simulink model "sg_2d_fir"  (Simulink 7.6)
settings: Solver=ode45  StartTime=0.0  StopTime=1600.0  RelTol=1e-3
undefined symbols (not defined in the file): gcbh, xlBlockLoadCallback, xlGetNormalizedPeriod, xlipgetpartsetting
libraries: xbsIndex_r4 x311, dspsrcs4 x6
(part 1 of 4)
settings Model: Creator=tbooth  LastModifiedBy=tawassne
settings OptimizationCC: InitFltsAndDblsToZero=on
settings DebuggingCC: SaveWithParameterizedLinksMsg=none  SignalResolutionControl=TryResolveAllWithWarning  MultiTaskDSMMsg=warning  MultiTaskCondExecSysMsg=none  StrictBusMsg=Warning
settings RTWCC: IncludeERTFirstTime=on
settings GRTTargetCC: TargetFcnLib=ansi_tfl_tmw.mat

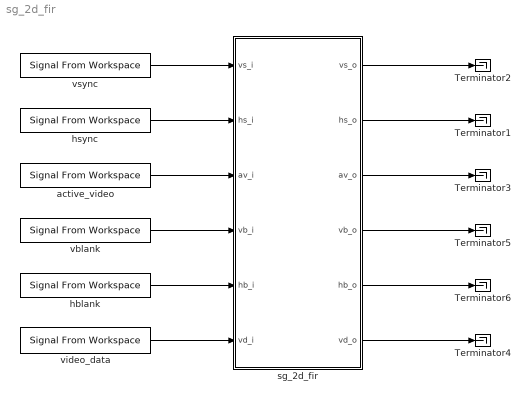
== system sg_2d_fir ==
  Terminator{1..6} (6 alike) : Terminator
  active_video : dspsrcs4/Signal From Workspace  SystemSampleTime=-1  X="[ones(1,90) zeros(1,10)  ]"  Ts=1  nsamps=1  OutputAfterFinalValue=Cyclic repetition  ignoreOrWarnInputAndFrameLengths=off
  hblank : dspsrcs4/Signal From Workspace  SystemSampleTime=-1  X=[ zeros(1,1) ones(1,99) ]  Ts=1  nsamps=1  OutputAfterFinalValue=Cyclic repetition  ignoreOrWarnInputAndFrameLengths=off
  hsync : dspsrcs4/Signal From Workspace  SystemSampleTime=-1  X=[ zeros(1,1) ones(1,99) ]  Ts=1  nsamps=1  OutputAfterFinalValue=Cyclic repetition  ignoreOrWarnInputAndFrameLengths=off
  sg_2d_fir : Subsystem
  vblank : dspsrcs4/Signal From Workspace  SystemSampleTime=-1  X=[ zeros(1,100) ones(1,900) ]  Ts=1  nsamps=1  OutputAfterFinalValue=Cyclic repetition  ignoreOrWarnInputAndFrameLengths=off
  video_data : dspsrcs4/Signal From Workspace  SystemSampleTime=-1  X=[repmat([10, 20],1,40),zeros(1,20), repmat([20,15],1,40) ,zeros(1,20)]  Ts=1  nsamps=1  OutputAfterFinalValue=Cyclic repetition  ignoreOrWarnInputAndFrameLengths=off
      link override From Workspace: OutputAfterFinalValue=Cyclic repetition
  vsync : dspsrcs4/Signal From Workspace  SystemSampleTime=-1  X=[ zeros(1,100) ones(1,900) ]  Ts=1  nsamps=1  OutputAfterFinalValue=Cyclic repetition  ignoreOrWarnInputAndFrameLengths=off
  wires:
  vsync/1 -> sg_2d_fir/1(vs_i)
  hsync/1 -> sg_2d_fir/2(hs_i)
  active_video/1 -> sg_2d_fir/3(av_i)
  sg_2d_fir/1(vs_o) -> Terminator2/1
  sg_2d_fir/2(hs_o) -> Terminator1/1
  sg_2d_fir/3(av_o) -> Terminator3/1
  sg_2d_fir/6(vd_o) -> Terminator4/1
  video_data/1 -> sg_2d_fir/6(vd_i)
  vblank/1 -> sg_2d_fir/4(vb_i)
  hblank/1 -> sg_2d_fir/5(hb_i)
  sg_2d_fir/4(vb_o) -> Terminator5/1
  sg_2d_fir/5(hb_o) -> Terminator6/1

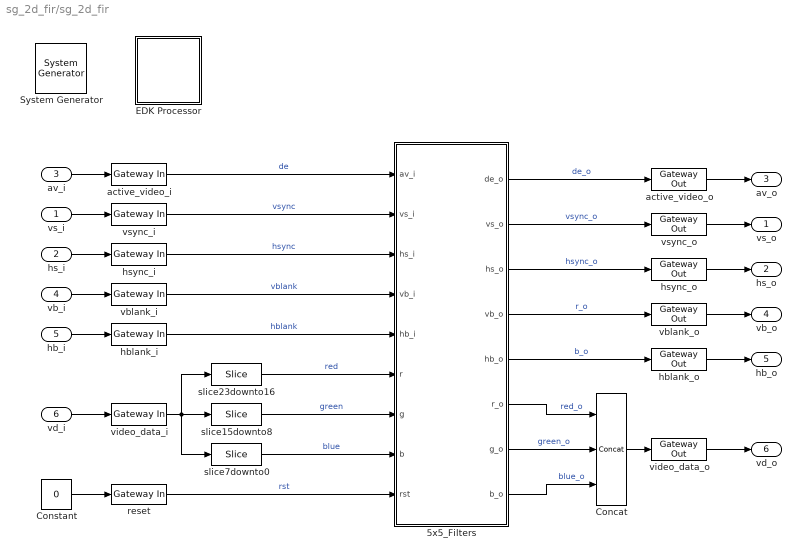
== system sg_2d_fir/sg_2d_fir ==
  vs_i : Inport
  hs_i : Inport  Port=2
  av_i : Inport  Port=3
  vb_i : Inport  Port=4
  hb_i : Inport  Port=5
  vd_i : Inport  Port=6
  " System Generator" : xbsIndex_r4/ System Generator  Tag=genX  SystemSampleTime=-1  xilinxfamily=spartan6  part=xc6slx150t  speed=-3  package=fgg676  synthesis_tool=XST  clock_wrapper=Clock Enables  directory=./sg_rgb_2d_fir_s6  proj_type=Project Navigator  Synth_file=XST Defaults  Impl_file=ISE Defaults  testbench=off  simulink_period=1  sysclk_period=10  dcm_input_clock_period=10  incr_netlist=off  trim_vbits=Everywhere in SubSystem  dbl_ovrd=According to Block Masks  core_generation=According to Block Masks  run_coregen=off  deprecated_control=off  eval_field=0  block_type=sysgen
      settings: block_version=11.4
  5x5_Filters : Subsystem
  Concat : xbsIndex_r4/Concat  num_inputs=3  dbl_ovrd=off  block_type=concat
  Constant : Constant  Value=0
  EDK Processor : Subsystem  LoadFcn=xlBlockLoadCallback(gcbh);  mask(Xilinx EDK Processor Block){mode=EDK pcore generation, xmp=, MemVisToProc=<qt bgcolor="#FFFFFF"><div><img src="C:/Program_Waj/Xilinx_13.1/ISE_DS/ISE/sysgen/data/images/registerminus.gif"> &lt;&lt;coef_update&gt;&gt;<br> <img src="C:/Program_Waj/Xilinx_13.1/ISE_DS/ISE/sysgen/data/images/parameters.gif"> Type : Fix_1_0<br> <img src="C:/Program_Waj/Xilinx_13.1/ISE_DS/ISE/sysgen/data/images/parameters.gif"> Addr : 0x80000800<br></div><div><img src="C:/Program_Waj/Xilinx_13.1/ISE_DS/ISE/sysgen/data/images/registerminus.gif"> &lt;&lt;coef_gain&gt;&gt;<br> <img src="C:/Program_Waj/Xilinx_13.1/ISE_DS/ISE/sysgen/data/images/parameters.gif"> Type : Fix_20_17<br> <img src="C:/Program_Waj/Xilinx_13.1/ISE_DS/ISE/sysgen/data/images/parameters.gif"> Addr : 0x80000804<br></div><div><img src="C:/Program_Waj/Xilinx_13.1/ISE_DS/ISE/sysgen/data/images/memoryminus.gif"> &lt;&lt;coef_buffer&gt;&gt;<br> <img src="C:/Program_Waj/Xilinx_13.1/ISE_DS/ISE/sysgen/data/images/parameters.gif"> Type : Fix_7_0<br> <img src="C:/Program_Waj/Xilinx_13.1/ISE_DS/ISE/sysgen/data/images/parameters.gif"> Addr : 0x80000000<br> <img src="C:/Program_Waj/Xilinx_13.1/ISE_DS/ISE/sysgen/data/images/parameters.gif"> Depth : 32<br></div></qt>, AvailableMemories=<empty>, portInterfaceTable={'exposed'=>[],'portdir'=>[],'portname'=>[],'shortname'=>[]}, bus_type_sgadvanced=, bus_type=PLB, baseaddr=0x80000000, baseaddr_lock_sgadvanced=, baseaddr_lock=off, dual_clock_sgadvanced=, dual_clock=on, reg_readback_sgadvanced=, reg_readback=on, ucf_file=, inheritDeviceType_sgadvanced=, inheritDeviceType=off, elf_file=, codebug_sgadvanced=, codebug=on, clock_name=plb, internalPortList={}, resetPolarity=0, memxtable={'mladdr'=>[0.00000000000000000,1.00000000000000000,-1.00000000000000000],'mlist'=>['sg_2d_fir/sg_2d_fir/5x5_Filters/coefficient_memory/From Register1','sg_2d_fir/sg_2d_fir/5x5_Filters/coefficient_memory/From Register','sg_2d_fir/sg_2d_fir/5x5_Filters/coefficient_memory/Shared Memory'],'mlname'=>['\\'coef_update\\'','\\'coef_gain\\'','\\'coef_buffer\\''],'mlstate'=>[1.00000000000000000,1.00000000000000000,1.00000000000000000]}, procinfo={}, memmapdirty=off, blockname=, xpsintstyle=default, has_advanced_control=0, sggui_pos=595,80,379,436, block_type=edkprocessor, block_version=2.7, sg_icon_stat=62,64,-1,-1,white,blue,0,07734,right,,[ ],[ ], sg_mask_display=|, sg_list_contents={'table'=>{'AvailableMemories'=>'popup(<empty>)'}}, sg_blockgui_xml=}
      mask sg_mask_display=|
      | fprintf('','COMMENT: begin icon graphics');
      | patch([0 62 62 0 0 ],[0 0 64 64 0 ],[0.77 0.82 0.91 ]);
      | plot([0 62 62 0 0 ],[0 0 64 64 0 ]);
      | patch([13.2 24.76 32.76 40.76 48.76 32.76 21.2 13.2 ],[40.88 40.88 48.88 40.88 48.88 48.88 48.88 40.88 ],[1 1 1 ]);
      | patch([21.2 32.76 24.76 13.2 21.2 ],[32.88 32.88 40.88 40.88 32.88 ],[0.931 0.946 0.973 ]);
      | patch([13.2 24.76 32.76 21.2 13.2 ],[24.88 24.88 32.88 32.88 24.88 ],[1 1 1 ]);
      | patch([21.2 48.76 40.76 32.76 24.76 13.2 21.2 ],[16.88 16.88 24.88 16.88 24.88 24.88 16.88 ],[0.931 0.946 0.973 ]);
      | fprintf('','COMMENT: end icon graphics');
      | fprintf('','COMMENT: begin icon text');
      | fprintf('','COMMENT: end icon text');
      mask prompts: mode "Configure Processor for"; xmp "XPS Project"; MemVisToProc ""; AvailableMemories "Available Memories"; portInterfaceTable ""; bus_type_sgadvanced ""; bus_type "Bus Type"; baseaddr "Base Address"; baseaddr_lock_sgadvanced ""; baseaddr_lock "Lock"; dual_clock_sgadvanced ""; dual_clock "Dual Clocks"; reg_readback_sgadvanced ""; reg_readback "Register Read-Back"; ucf_file "Constraint File"; inheritDeviceType_sgadvanced ""; inheritDeviceType "Inherit Device Type"; elf_file "Initial Program"; codebug_sgadvanced ""; codebug "Enable Co-Debug with Xilinx SDK (Beta)"; clock_name ""; internalPortList ""; resetPolarity ""; memxtable ""; procinfo ""; memmapdirty ""; blockname ""; xpsintstyle ""; has_advanced_control ""; sggui_pos ""; block_type ""; block_version ""; sg_icon_stat ""; sg_mask_display ""; sg_list_contents ""; sg_blockgui_xml ""
      mask help: Xilinx EDK Processor
      mask init:
      | try
      |   tmp_gcb = gcb;
      |   tmp_gcbh = gcbh;
      |   if (strcmp('SysGenIndex',get_param(bdroot(tmp_gcbh),'tag')) && ~isempty(regexp(bdroot(tmp_gcb), '^xbs', 'once')))
      |     return;
      |   end;
      |   xlMungeMaskParams;
      | 
      |   block_type='edkprocessor';
      | 
      |   serialized_declarations = '{''block_type''=>''String''}';
      |   xledkprocessor_init();
      |   ptable_ = xlblockprep(get_param(tmp_gcb, 'MaskWSVariables'));
      |   try
      |     xlBlockMoveCallback(tmp_gcbh);
      |   catch 
      |      clear global xl_updateicon_recursion_guard;
      |   end;
      | catch
      |   global dbgsysgen;
      |   if(~isempty(dbgsysgen) && dbgsysgen)
      |     e = regexprep(lasterr, '\n', '\nError: ');
      |     disp(['Error: While running MaskInit code on block ' tmp_gcb ': ' e]);
      |     error(e);
      |   end
      | end
      settings: CopyFcn=xlProcBlockCopyCallback(gcbh);xlBlockMoveCallback(gcbh);  DeleteFcn=xlDestroyGui(gcbh);  ModelCloseFcn=xlDestroyGui(gcbh);  PreSaveFcn=xlBlockPreSaveCallback(gcbh);  PostSaveFcn=xlBlockPostSaveCallback(gcbh);  DestroyFcn=xlDestroyGui(gcbh);  OpenFcn=bh=gcbh;xlProcBlockCallbacks('populatesharedmemorylistbox',bh);xlOpenGui(bh, 'edkprocessor_gui.xml', @xlProcBlockEnablement, @xlProcBlockAction);  CloseFcn=xlDestroyGui(gcbh);  MoveFcn=xlBlockMoveCallback(gcbh);
      mask Help: eval('');xlDoc('-book','sysgen','-topic','EDK_Processor');
      mask StyleString: popup(EDK pcore generation|HDL netlisting),edit,edit,edit,edit,edit,popup(AXI|PLB),edit,edit,checkbox,edit,checkbox,edit,checkbox,edit,edit,checkbox,edit,edit,checkbox,edit,edit,edit,edit,edit,edit,edit,edit,edit,edit,edit,edit,edit,edit,edit,edit
      mask Display:
      | fprintf('','COMMENT: begin icon graphics');
      | patch([0 62 62 0 0 ],[0 0 64 64 0 ],[0.77 0.82 0.91 ]);
      | plot([0 62 62 0 0 ],[0 0 64 64 0 ]);
      | patch([13.2 24.76 32.76 40.76 48.76 32.76 21.2 13.2 ],[40.88 40.88 48.88 40.88 48.88 48.88 48.88 40.88 ],[1 1 1 ]);
      | patch([21.2 32.76 24.76 13.2 21.2 ],[32.88 32.88 40.88 40.88 32.88 ],[0.931 0.946 0.973 ]);
      | patch([13.2 24.76 32.76 21.2 13.2 ],[24.88 24.88 32.88 32.88 24.88 ],[1 1 1 ]);
      | patch([21.2 48.76 40.76 32.76 24.76 13.2 21.2 ],[16.88 16.88 24.88 16.88 24.88 24.88 16.88 ],[0.931 0.946 0.973 ]);
      | fprintf('','COMMENT: end icon graphics');
      | fprintf('','COMMENT: begin icon text');
      | disp('');
      | 
      | fprintf('','COMMENT: end icon text');
  active_video_i : xbsIndex_r4/Gateway In  gui_display_data_type=Fixed-point  arith_type=Unsigned  n_bits=1  bin_pt=0  preci_type=Single  exp_width=8  frac_width=24  quantization="Round  (unbiased: +/- Inf)"  overflow=Saturate  period=1  dbl_ovrd=off  timing_constraint=None  locs_specified=off  LOCs={}  hdl_port=on  block_type=gatewayin
      settings: infoedit="Gateway in block.  Converts inputs of type Simulink integer, double and fixed point to  Xilinx fixed point type.<P><P>Hardware notes:  In hardware these blocks become top level input ports."  xl_area=[0, 0, 0, 0, 0, 0, 0]  block_version=VER_STRING_GOES_HERE
  active_video_o : xbsIndex_r4/Gateway Out  hdl_port=on  timing_constraint=None  locs_specified=off  LOCs={}  block_type=gatewayout
      settings: infoedit="Gateway out block.  Converts Xilinx fixed point inputs into ouputs of type Simulink integer, double, or fixed point.<P><P>Hardware notes:  In hardware these blocks become top level output ports or are discarded, depending on how they are configured."  xl_area=[0, 0, 0, 0, 0, 0, 0]  block_version=VER_STRING_GOES_HERE
  hblank_i : xbsIndex_r4/Gateway In  gui_display_data_type=Fixed-point  arith_type=Unsigned  n_bits=1  bin_pt=0  preci_type=Single  exp_width=8  frac_width=24  quantization="Round  (unbiased: +/- Inf)"  overflow=Saturate  period=1  dbl_ovrd=off  timing_constraint=None  locs_specified=off  LOCs={}  hdl_port=on  block_type=gatewayin
      settings: infoedit="Gateway in block.  Converts inputs of type Simulink integer, double and fixed point to  Xilinx fixed point type.<P><P>Hardware notes:  In hardware these blocks become top level input ports."  xl_area=[0, 0, 0, 0, 0, 0, 0]  block_version=VER_STRING_GOES_HERE
  hblank_o : xbsIndex_r4/Gateway Out  hdl_port=on  timing_constraint=None  locs_specified=off  LOCs={}  block_type=gatewayout
      settings: infoedit="Gateway out block.  Converts Xilinx fixed point inputs into ouputs of type Simulink integer, double, or fixed point.<P><P>Hardware notes:  In hardware these blocks become top level output ports or are discarded, depending on how they are configured."  xl_area=[0, 0, 0, 0, 0, 0, 0]  block_version=VER_STRING_GOES_HERE
  hsync_i : xbsIndex_r4/Gateway In  gui_display_data_type=Fixed-point  arith_type=Unsigned  n_bits=1  bin_pt=0  preci_type=Single  exp_width=8  frac_width=24  quantization="Round  (unbiased: +/- Inf)"  overflow=Saturate  period=1  dbl_ovrd=off  timing_constraint=None  locs_specified=off  LOCs={}  hdl_port=on  block_type=gatewayin
      settings: infoedit="Gateway in block.  Converts inputs of type Simulink integer, double and fixed point to  Xilinx fixed point type.<P><P>Hardware notes:  In hardware these blocks become top level input ports."  xl_area=[0, 0, 0, 0, 0, 0, 0]  block_version=VER_STRING_GOES_HERE
  hsync_o : xbsIndex_r4/Gateway Out  hdl_port=on  timing_constraint=None  locs_specified=off  LOCs={}  block_type=gatewayout
      settings: infoedit="Gateway out block.  Converts Xilinx fixed point inputs into ouputs of type Simulink integer, double, or fixed point.<P><P>Hardware notes:  In hardware these blocks become top level output ports or are discarded, depending on how they are configured."  xl_area=[0, 0, 0, 0, 0, 0, 0]  block_version=VER_STRING_GOES_HERE
  reset : xbsIndex_r4/Gateway In  gui_display_data_type=Fixed-point  arith_type=Unsigned  n_bits=1  bin_pt=0  preci_type=Single  exp_width=8  frac_width=24  quantization="Round  (unbiased: +/- Inf)"  overflow=Saturate  period=1  dbl_ovrd=off  timing_constraint=None  locs_specified=off  LOCs={}  hdl_port=on  block_type=gatewayin
      settings: infoedit="Gateway in block.  Converts inputs of type Simulink integer, double and fixed point to  Xilinx fixed point type.<P><P>Hardware notes:  In hardware these blocks become top level input ports."
  slice15downto8 : xbsIndex_r4/Slice  nbits=8  boolean_output=off  mode=Lower Bit Location + Width  bit1=0  base1=MSB of Input  bit0=8  base0=LSB of Input  dbl_ovrd=off  block_type=slice
  slice23downto16 : xbsIndex_r4/Slice  nbits=8  boolean_output=off  mode=Lower Bit Location + Width  bit1=0  base1=MSB of Input  bit0=16  base0=LSB of Input  dbl_ovrd=off  block_type=slice
  slice7downto0 : xbsIndex_r4/Slice  nbits=8  boolean_output=off  mode=Lower Bit Location + Width  bit1=0  base1=MSB of Input  bit0=0  base0=LSB of Input  dbl_ovrd=off  block_type=slice
  vblank_i : xbsIndex_r4/Gateway In  gui_display_data_type=Fixed-point  arith_type=Unsigned  n_bits=1  bin_pt=0  preci_type=Single  exp_width=8  frac_width=24  quantization="Round  (unbiased: +/- Inf)"  overflow=Saturate  period=1  dbl_ovrd=off  timing_constraint=None  locs_specified=off  LOCs={}  hdl_port=on  block_type=gatewayin
      settings: infoedit="Gateway in block.  Converts inputs of type Simulink integer, double and fixed point to  Xilinx fixed point type.<P><P>Hardware notes:  In hardware these blocks become top level input ports."  xl_area=[0, 0, 0, 0, 0, 0, 0]  block_version=VER_STRING_GOES_HERE
  vblank_o : xbsIndex_r4/Gateway Out  hdl_port=on  timing_constraint=None  locs_specified=off  LOCs={}  block_type=gatewayout
      settings: infoedit="Gateway out block.  Converts Xilinx fixed point inputs into ouputs of type Simulink integer, double, or fixed point.<P><P>Hardware notes:  In hardware these blocks become top level output ports or are discarded, depending on how they are configured."  xl_area=[0, 0, 0, 0, 0, 0, 0]  block_version=VER_STRING_GOES_HERE
  video_data_i : xbsIndex_r4/Gateway In  gui_display_data_type=Fixed-point  arith_type=Unsigned  n_bits=24  bin_pt=0  preci_type=Single  exp_width=8  frac_width=24  quantization="Round  (unbiased: +/- Inf)"  overflow=Saturate  period=1  dbl_ovrd=off  timing_constraint=None  locs_specified=off  LOCs={}  hdl_port=on  block_type=gatewayin
      settings: infoedit="Gateway in block.  Converts inputs of type Simulink integer, double and fixed point to  Xilinx fixed point type.<br><br>Hardware notes:  In hardware these blocks become top level input ports."  xl_area=[0, 0, 0, 0, 0, 0, 0]  block_version=VER_STRING_GOES_HERE
  video_data_o : xbsIndex_r4/Gateway Out  hdl_port=on  timing_constraint=None  locs_specified=off  LOCs={}  block_type=gatewayout
      settings: infoedit="Gateway out block.  Converts Xilinx fixed point inputs into ouputs of type Simulink integer, double, or fixed point.<P><P>Hardware notes:  In hardware these blocks become top level output ports or are discarded, depending on how they are configured."  xl_area=[0, 0, 0, 0, 0, 0, 0]  block_version=VER_STRING_GOES_HERE
  vsync_i : xbsIndex_r4/Gateway In  gui_display_data_type=Fixed-point  arith_type=Unsigned  n_bits=1  bin_pt=0  preci_type=Single  exp_width=8  frac_width=24  quantization="Round  (unbiased: +/- Inf)"  overflow=Saturate  period=1  dbl_ovrd=off  timing_constraint=None  locs_specified=off  LOCs={}  hdl_port=on  block_type=gatewayin
      settings: infoedit="Gateway in block.  Converts inputs of type Simulink integer, double and fixed point to  Xilinx fixed point type.<P><P>Hardware notes:  In hardware these blocks become top level input ports."  xl_area=[0, 0, 0, 0, 0, 0, 0]  block_version=VER_STRING_GOES_HERE
  vsync_o : xbsIndex_r4/Gateway Out  hdl_port=on  timing_constraint=None  locs_specified=off  LOCs={}  block_type=gatewayout
      settings: infoedit="Gateway out block.  Converts Xilinx fixed point inputs into ouputs of type Simulink integer, double, or fixed point.<P><P>Hardware notes:  In hardware these blocks become top level output ports or are discarded, depending on how they are configured."  xl_area=[0, 0, 0, 0, 0, 0, 0]  block_version=VER_STRING_GOES_HERE
  vs_o : Outport
  hs_o : Outport  Port=2
  av_o : Outport  Port=3
  vb_o : Outport  Port=4
  hb_o : Outport  Port=5
  vd_o : Outport  Port=6
  wires:
  5x5_Filters/1(de_o) -> active_video_o/1  "de_o"
  5x5_Filters/2(vs_o) -> vsync_o/1  "vsync_o"
  5x5_Filters/3(hs_o) -> hsync_o/1  "hsync_o"
  Constant/1 -> reset/1
  hsync_i/1 -> 5x5_Filters/3(hs_i)  "hsync"
  active_video_i/1 -> 5x5_Filters/1(av_i)  "de"
  vsync_i/1 -> 5x5_Filters/2(vs_i)  "vsync"
  av_i/1 -> active_video_i/1
  vs_i/1 -> vsync_i/1
  hs_i/1 -> hsync_i/1
  vd_i/1 -> video_data_i/1
  active_video_o/1 -> av_o/1
  vsync_o/1 -> vs_o/1
  hsync_o/1 -> hs_o/1
  video_data_o/1 -> vd_o/1
  Concat/1 -> video_data_o/1
  slice23downto16/1 -> 5x5_Filters/6(r)  "red"
  reset/1 -> 5x5_Filters/9(rst)  "rst"
  vblank_o/1 -> vb_o/1
  hblank_o/1 -> hb_o/1
  vb_i/1 -> vblank_i/1
  hb_i/1 -> hblank_i/1
  5x5_Filters/4(vb_o) -> vblank_o/1  "r_o"
  5x5_Filters/5(hb_o) -> hblank_o/1  "b_o"
  vblank_i/1 -> 5x5_Filters/4(vb_i)  "vblank"
  hblank_i/1 -> 5x5_Filters/5(hb_i)  "hblank"
  video_data_i/1 -> slice7downto0/1, slice23downto16/1, slice15downto8/1
  slice15downto8/1 -> 5x5_Filters/7(g)  "green"
  slice7downto0/1 -> 5x5_Filters/8(b)  "blue"
  5x5_Filters/7(g_o) -> Concat/2  "green_o"
  5x5_Filters/8(b_o) -> Concat/3  "blue_o"
  5x5_Filters/6(r_o) -> Concat/1  "red_o"

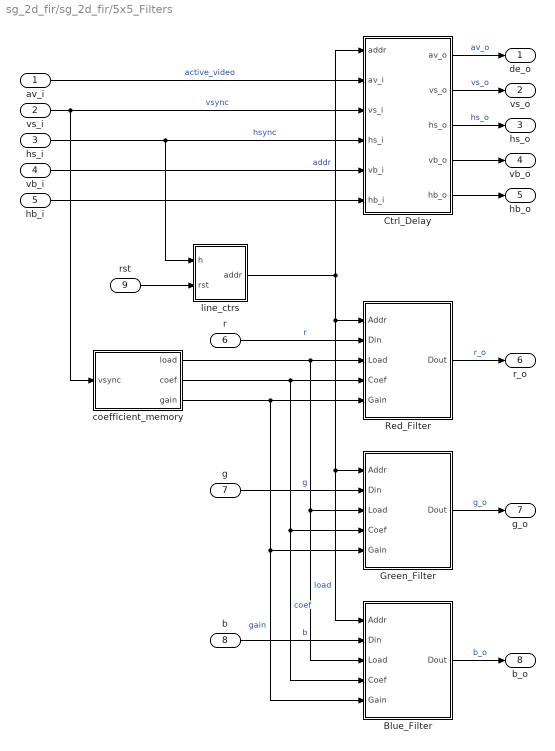
== system sg_2d_fir/sg_2d_fir/5x5_Filters ==
  av_i : Inport
  vs_i : Inport  Port=2
  hs_i : Inport  Port=3
  vb_i : Inport  Port=4
  hb_i : Inport  Port=5
  r : Inport  Port=6
  g : Inport  Port=7
  b : Inport  Port=8
  rst : Inport  Port=9
  Blue_Filter : Subsystem
  Ctrl_Delay : Subsystem
  Green_Filter : Subsystem
  Red_Filter : Subsystem
  coefficient_memory : Subsystem  mask{width=7, bin_pt=0, g_width=20, g_bin_pt=17, period=1}
      mask prompts: width "Coefficient Width"; bin_pt "Coefficient Binary Point"; g_width "Gain Width"; g_bin_pt "Gain Binary Point"; period "Sample Period"
      mask init:
      | %work around until plb initialization can use mask variables
      | 
      | c_width = sprintf('%d',width);
      | c_bin_pt = sprintf('%d',bin_pt);
      | c_g_width = sprintf('%d',g_width);
      | c_g_bin_pt = sprintf('%d',g_bin_pt);
      | 
      | blockPath = gcs;
      | set_param([blockPath '/coefficient_memory/Shared Memory'],'n_bits',c_width);
      | set_param([blockPath '/coefficient_memory/Shared Memory'],'bin_pt',c_bin_pt);
      | 
      | set_param([blockPath '/coefficient_memory/From Register'],'n_bits',c_g_width);
      | set_param([blockPath '/coefficient_memory/From Register'],'bin_pt',c_g_bin_pt);
  line_ctrs : Subsystem
  de_o : Outport
  vs_o : Outport  Port=2
  hs_o : Outport  Port=3
  vb_o : Outport  Port=4
  hb_o : Outport  Port=5
  r_o : Outport  Port=6
  g_o : Outport  Port=7
  b_o : Outport  Port=8
  wires:
  r/1 -> Red_Filter/2(Din)  "r"
  coefficient_memory/1(load) -> Red_Filter/3(Load), Green_Filter/3(Load), Blue_Filter/3(Load)  "load"
  coefficient_memory/2(coef) -> Red_Filter/4(Coef), Green_Filter/4(Coef), Blue_Filter/4(Coef)  "coef"
  Red_Filter/1(Dout) -> r_o/1  "r_o"
  coefficient_memory/3(gain) -> Red_Filter/5(Gain), Green_Filter/5(Gain), Blue_Filter/5(Gain)  "gain"
  hs_i/1 -> line_ctrs/1(h), Ctrl_Delay/4(hs_i)  "hsync"
  line_ctrs/1(addr) -> Ctrl_Delay/1(addr), Red_Filter/1(Addr), Green_Filter/1(Addr), Blue_Filter/1(Addr)  "addr"
  vs_i/1 -> Ctrl_Delay/3(vs_i), coefficient_memory/1(vsync)  "vsync"
  av_i/1 -> Ctrl_Delay/2(av_i)  "active_video"
  Ctrl_Delay/3(hs_o) -> hs_o/1  "hs_o"
  Ctrl_Delay/2(vs_o) -> vs_o/1  "vs_o"
  Ctrl_Delay/1(av_o) -> de_o/1  "av_o"
  g/1 -> Green_Filter/2(Din)  "g"
  Green_Filter/1(Dout) -> g_o/1  "g_o"
  b/1 -> Blue_Filter/2(Din)  "b"
  Blue_Filter/1(Dout) -> b_o/1  "b_o"
  rst/1 -> line_ctrs/2(rst)
  Ctrl_Delay/5(hb_o) -> hb_o/1
  Ctrl_Delay/4(vb_o) -> vb_o/1
  vb_i/1 -> Ctrl_Delay/5(vb_i)
  hb_i/1 -> Ctrl_Delay/6(hb_i)

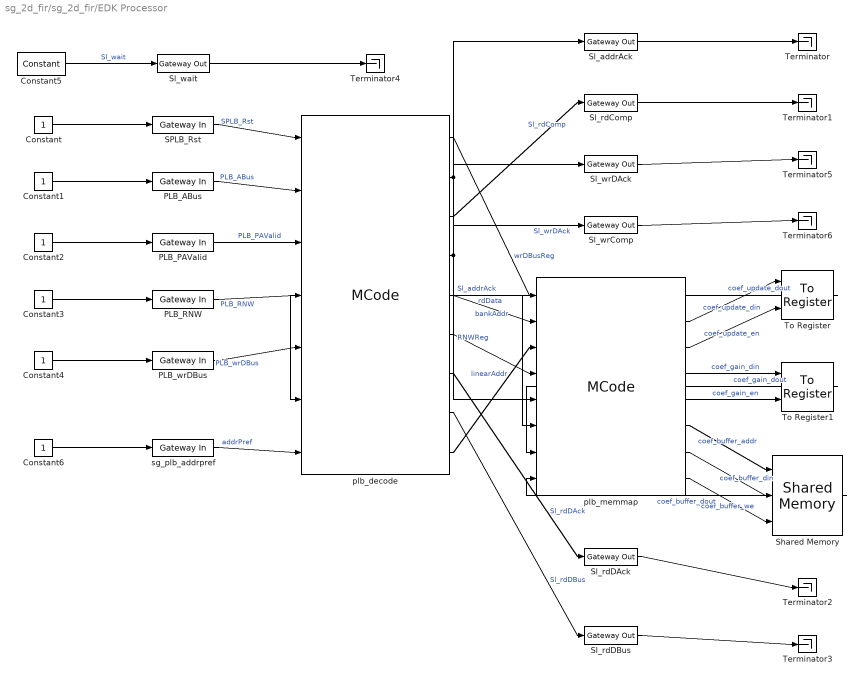
== system sg_2d_fir/sg_2d_fir/EDK Processor ==
  Constant{,1..4,6} (6 alike) : Constant
  Constant5 : xbsIndex_r4/Constant  const=0  gui_display_data_type=Fixed-point  arith_type=Unsigned  n_bits=1  bin_pt=0  preci_type=Single  exp_width=8  frac_width=24  explicit_period=on  period=xlGetNormalizedPeriod()  equ=P=C  opselect=C  inp2=PCIN>>17  opr=+  inp1=P  carry=CIN  dbl_ovrd=off  block_type=constant
  PLB_ABus : xbsIndex_r4/Gateway In  gui_display_data_type=Fixed-point  arith_type=Unsigned  n_bits=32  bin_pt=0  preci_type=Single  exp_width=8  frac_width=24  quantization="Round  (unbiased: +/- Inf)"  overflow=Saturate  period=xlGetNormalizedPeriod()  dbl_ovrd=off  timing_constraint=None  locs_specified=off  LOCs={}  hdl_port=on  block_type=gatewayin
      settings: infoedit="Gateway in block.  Converts inputs of type Simulink integer, double and fixed point to  Xilinx fixed point or floating-point data type.<br><br>Hardware notes:  In hardware these blocks become top level input ports."  sginterface={'Xilinx'=>{'jtaghwcosim'=>{'non_memory_mapped_port'=>'PLB_ABus'}},'iopad'=>{'constraint'=>'#'}}
  PLB_PAValid : xbsIndex_r4/Gateway In  gui_display_data_type=Fixed-point  arith_type=Unsigned  n_bits=1  bin_pt=0  preci_type=Single  exp_width=8  frac_width=24  quantization="Round  (unbiased: +/- Inf)"  overflow=Saturate  period=xlGetNormalizedPeriod()  dbl_ovrd=off  timing_constraint=None  locs_specified=off  LOCs={}  hdl_port=on  block_type=gatewayin
      settings: infoedit="Gateway in block.  Converts inputs of type Simulink integer, double and fixed point to  Xilinx fixed point or floating-point data type.<br><br>Hardware notes:  In hardware these blocks become top level input ports."  sginterface={'Xilinx'=>{'jtaghwcosim'=>{'non_memory_mapped_port'=>'PLB_PAValid'}},'iopad'=>{'constraint'=>'#'}}
  PLB_RNW : xbsIndex_r4/Gateway In  gui_display_data_type=Fixed-point  arith_type=Unsigned  n_bits=1  bin_pt=0  preci_type=Single  exp_width=8  frac_width=24  quantization="Round  (unbiased: +/- Inf)"  overflow=Saturate  period=xlGetNormalizedPeriod()  dbl_ovrd=off  timing_constraint=None  locs_specified=off  LOCs={}  hdl_port=on  block_type=gatewayin
      settings: infoedit="Gateway in block.  Converts inputs of type Simulink integer, double and fixed point to  Xilinx fixed point or floating-point data type.<br><br>Hardware notes:  In hardware these blocks become top level input ports."  sginterface={'Xilinx'=>{'jtaghwcosim'=>{'non_memory_mapped_port'=>'PLB_RNW'}},'iopad'=>{'constraint'=>'#'}}
  PLB_wrDBus : xbsIndex_r4/Gateway In  gui_display_data_type=Fixed-point  arith_type=Unsigned  n_bits=32  bin_pt=0  preci_type=Single  exp_width=8  frac_width=24  quantization="Round  (unbiased: +/- Inf)"  overflow=Saturate  period=xlGetNormalizedPeriod()  dbl_ovrd=off  timing_constraint=None  locs_specified=off  LOCs={}  hdl_port=on  block_type=gatewayin
      settings: infoedit="Gateway in block.  Converts inputs of type Simulink integer, double and fixed point to  Xilinx fixed point or floating-point data type.<br><br>Hardware notes:  In hardware these blocks become top level input ports."  sginterface={'Xilinx'=>{'jtaghwcosim'=>{'non_memory_mapped_port'=>'PLB_wrDBus'}},'iopad'=>{'constraint'=>'#'}}
  SPLB_Rst : xbsIndex_r4/Gateway In  gui_display_data_type=Fixed-point  arith_type=Unsigned  n_bits=1  bin_pt=0  preci_type=Single  exp_width=8  frac_width=24  quantization="Round  (unbiased: +/- Inf)"  overflow=Saturate  period=xlGetNormalizedPeriod()  dbl_ovrd=off  timing_constraint=None  locs_specified=off  LOCs={}  hdl_port=on  block_type=gatewayin
      settings: infoedit="Gateway in block.  Converts inputs of type Simulink integer, double and fixed point to  Xilinx fixed point or floating-point data type.<br><br>Hardware notes:  In hardware these blocks become top level input ports."  sginterface={'Xilinx'=>{'jtaghwcosim'=>{'non_memory_mapped_port'=>'SPLB_Rst'}},'iopad'=>{'constraint'=>'#'}}
  Shared Memory : xbsIndex_r4/Shared Memory  shared_memory_name='coef_buffer'  depth=32  ownership=Owned and Initialized Elsewhere  initVector=sin(pi*(0:15)/16)  en=off  mutex=Unprotected  mode=Read and Write  write_mode=Read Before Write  time_out=0  latency=1  explicit_data_type=off  gui_display_data_type=Fixed-point  arith_type="Signed  (2's comp)"  n_bits=7  bin_pt=0  preci_type=Single  implementation=Block RAM  use_rpm=off  block_type=shmem
      settings: AttributesFormatString=<< %<shared_memory_name> >>
  Sl_addrAck : xbsIndex_r4/Gateway Out  hdl_port=on  timing_constraint=None  locs_specified=off  LOCs={}  block_type=gatewayout
      settings: infoedit="Gateway out block.  Converts Xilinx fixed point or floating-point type inputs into ouputs of type Simulink integer, double, or fixed point.<br><br>Hardware notes:  In hardware these blocks become top level output ports or are discarded, depending on how they are configured."  sginterface={'Xilinx'=>{'jtaghwcosim'=>{'non_memory_mapped_port'=>'Sl_addrAck'}},'iopad'=>{'constraint'=>'#'}}
  Sl_rdComp : xbsIndex_r4/Gateway Out  hdl_port=on  timing_constraint=None  locs_specified=off  LOCs={}  block_type=gatewayout
      settings: infoedit="Gateway out block.  Converts Xilinx fixed point or floating-point type inputs into ouputs of type Simulink integer, double, or fixed point.<br><br>Hardware notes:  In hardware these blocks become top level output ports or are discarded, depending on how they are configured."  sginterface={'Xilinx'=>{'jtaghwcosim'=>{'non_memory_mapped_port'=>'Sl_rdComp'}},'iopad'=>{'constraint'=>'#'}}
  Sl_rdDAck : xbsIndex_r4/Gateway Out  hdl_port=on  timing_constraint=None  locs_specified=off  LOCs={}  block_type=gatewayout
      settings: infoedit="Gateway out block.  Converts Xilinx fixed point or floating-point type inputs into ouputs of type Simulink integer, double, or fixed point.<br><br>Hardware notes:  In hardware these blocks become top level output ports or are discarded, depending on how they are configured."  sginterface={'Xilinx'=>{'jtaghwcosim'=>{'non_memory_mapped_port'=>'Sl_rdDAck'}},'iopad'=>{'constraint'=>'#'}}
  Sl_rdDBus : xbsIndex_r4/Gateway Out  hdl_port=on  timing_constraint=None  locs_specified=off  LOCs={}  block_type=gatewayout
      settings: infoedit="Gateway out block.  Converts Xilinx fixed point or floating-point type inputs into ouputs of type Simulink integer, double, or fixed point.<br><br>Hardware notes:  In hardware these blocks become top level output ports or are discarded, depending on how they are configured."  sginterface={'Xilinx'=>{'jtaghwcosim'=>{'non_memory_mapped_port'=>'Sl_rdDBus'}},'iopad'=>{'constraint'=>'#'}}
  Sl_wait : xbsIndex_r4/Gateway Out  hdl_port=on  timing_constraint=None  locs_specified=off  LOCs={}  block_type=gatewayout
      settings: infoedit="Gateway out block.  Converts Xilinx fixed point or floating-point type inputs into ouputs of type Simulink integer, double, or fixed point.<br><br>Hardware notes:  In hardware these blocks become top level output ports or are discarded, depending on how they are configured."  sginterface={'Xilinx'=>{'jtaghwcosim'=>{'non_memory_mapped_port'=>'Sl_wait'}},'iopad'=>{'constraint'=>'#'}}
  Sl_wrComp : xbsIndex_r4/Gateway Out  hdl_port=on  timing_constraint=None  locs_specified=off  LOCs={}  block_type=gatewayout
      settings: infoedit="Gateway out block.  Converts Xilinx fixed point or floating-point type inputs into ouputs of type Simulink integer, double, or fixed point.<br><br>Hardware notes:  In hardware these blocks become top level output ports or are discarded, depending on how they are configured."  sginterface={'Xilinx'=>{'jtaghwcosim'=>{'non_memory_mapped_port'=>'Sl_wrComp'}},'iopad'=>{'constraint'=>'#'}}
  Sl_wrDAck : xbsIndex_r4/Gateway Out  hdl_port=on  timing_constraint=None  locs_specified=off  LOCs={}  block_type=gatewayout
      settings: infoedit="Gateway out block.  Converts Xilinx fixed point or floating-point type inputs into ouputs of type Simulink integer, double, or fixed point.<br><br>Hardware notes:  In hardware these blocks become top level output ports or are discarded, depending on how they are configured."  sginterface={'Xilinx'=>{'jtaghwcosim'=>{'non_memory_mapped_port'=>'Sl_wrDAck'}},'iopad'=>{'constraint'=>'#'}}
  Terminator{,1..6} (7 alike) : Terminator
  To Register : xbsIndex_r4/To Register  shared_memory_name='coef_update'  init=0  ownership=Owned and initialized elsewhere  explicit_data_type=on  gui_display_data_type=Fixed-point  arith_type=Unsigned  n_bits=1  bin_pt=0  preci_type=Single  dbl_ovrd=off  block_type=toreg
      settings: AttributesFormatString=<< %<shared_memory_name> >>  infoedit="Register block that writes data to a shared memory register.  Delay of one sample period."
  To Register1 : xbsIndex_r4/To Register  shared_memory_name='coef_gain'  init=0  ownership=Owned and initialized elsewhere  explicit_data_type=on  gui_display_data_type=Fixed-point  arith_type=Unsigned  n_bits=20  bin_pt=17  preci_type=Single  dbl_ovrd=off  block_type=toreg
      settings: AttributesFormatString=<< %<shared_memory_name> >>  infoedit="Register block that writes data to a shared memory register.  Delay of one sample period."
  plb_decode : xbsIndex_r4/MCode  mfname=xlmax  explicit_period=off  period=1  dbl_ovrd=off  enable_stdout=off  enable_debug=off  mfilecontent=|  suppress_output=on  defparams={}  hide_port_list={}  block_type=mcode
      | function [wrDBusReg, addrAck, rdComp, wrDAck, bankAddr, RNWReg, rdDAck, rdDBus, linearAddr] = plb_bus_decode(plbRst, plbABus, plbPAValid, plbRNW, plbWrDBus, rdData, addrPref)
      | 
      | % constant variables (TODO: should pass from outside)
      | ADDRPREF_LEN = 20;
      | BANKADDR_LEN = 2;
      | LINEARADDR_LEN = 8;
      | ABUS_LEN = 32;
      | DBUS_LEN = 32;
      | 
      | % declare and initialize persistent variables
      | % register input bus signals
      | persistent plbRstReg_, plbRstReg_ = xl_state(0, {xlBoolean});
      | persistent plbABusReg_, plbABusReg_ = xl_state(0, {xlUnsigned, ABUS_LEN, 0});
      | persistent plbPAValidReg_, plbPAValidReg_ = xl_state(0, {xlBoolean});
      | persistent plbRNWReg_, plbRNWReg_ = xl_state(0, {xlUnsigned, 1, 0});
      | persistent plbWrDBusReg_, plbWrDBusReg_ = xl_state(0, {xlUnsigned, DBUS_LEN, 0});
      | 
      | % ===== rest of the outputs =====
      | 
      | bankAddr   = xl_slice(plbABusReg_, 2+BANKADDR_LEN+LINEARADDR_LEN-1, 2+LINEARADDR_LEN);
      | linearAddr = xl_slice(plbABusReg_, 2+LINEARADDR_LEN-1, 2);
      | RNWReg = plbRNWReg_;
      | wrDBusReg = plbWrDBusReg_;
      | 
      | % ===== p_select =====
      | 
      | % register PAValid
      | persistent aValidReg, aValidReg = xl_state(0, {xlBoolean});
      | aValidReg = plbPAValidReg_;
      | 
      | % extract and register the address prefix
      | addrPref_in = xl_slice(plbABusReg_, xl_nbits(plbABusReg_)-1, xl_nbits(plbABusReg_)-ADDRPREF_LEN);
      | if addrPref_in == addrPref
      |     ps1 = true;
      | else 
      |     ps1 = false;
      | end 
      | 
      | persistent ps1Reg, ps1Reg = xl_state(0, ps1);
      | ps1Reg = ps1;
      | 
      | ps = xl_and(ps1Reg, aValidReg);
      | 
      | % ===== addrAck =====
      | 
      | % register ps
      | persistent psReg, psReg = xl_state(0, ps);
      | 
      | addrAck = xfix({xlUnsigned, 1, 0}, xl_and(xl_not(plbRstReg_), ps, xl_not(psReg)));
      | 
      | psReg = ps;
      | 
      | % ===== rdComp, rd/wr DAck =====
      |  
      | rdComp1 = xfix({xlUnsigned, 1, 0}, xl_and(addrAck, RNWReg));
      | 
      | NUM_rdCompDelay = 3;
      | persistent rdCompDelay, rdCompDelay = xl_state(zeros(1, NUM_rdCompDelay), rdComp1, NUM_rdCompDelay);
      | rdComp2 = rdCompDelay.back;
      | rdCompDelay.push_front_pop_back(rdComp1);
      | 
      | persistent rdCompReg, rdCompReg = xl_state(0, rdComp1);
      | rdComp = rdCompReg;
      | rdCompReg = rdComp2;
      | 
      | persistent rdDAckReg, rdDAckReg = xl_state(0, rdComp1);
      | rdDAck = rdDAckReg;
      | rdDAckReg = rdComp;
      | 
      | persistent wrDAckReg, wrDAckReg = xl_state(0, addrAck);
      | wrDAck = wrDAckReg;
      | wrDAckReg = xl_and(addrAck, xl_not(RNWReg));
      | 
      | % ===== rdDBus =====
      | 
      | rdSel = xl_or(rdComp2, rdComp);
      | 
      | if rdSel == 1
      |     rdDBus1 = rdData;
      | else
      |     rdDBus1 = 0;
      | end % if
      | 
      | persistent rdDBusReg, rdDBusReg = xl_state(0, rdDBus1);
      | rdDBus = rdDBusReg;
      | rdDBusReg = rdDBus1;
      | 
      | % rdDBus = xl_concat(rdDBus32, rdDBus32);
      | % rdDBus = rdDBus32;
      | 
      | % ===== update the persistent variables =====
      | 
      | plbRstReg_ = plbRst;
      | plbABusReg_ = plbABus;
      | plbPAValidReg_ = plbPAValid;
      | plbRNWReg_ = plbRNW;
      | plbWrDBusReg_ = xl_slice(plbWrDBus, DBUS_LEN-1, 0);
  plb_memmap : xbsIndex_r4/MCode  mfname=xlmax  explicit_period=off  period=1  dbl_ovrd=off  enable_stdout=off  enable_debug=off  mfilecontent=|  suppress_output=on  defparams={}  hide_port_list={}  block_type=mcode
      | function [read_bank_out, sm_coef_update_din, sm_coef_update_en, sm_coef_gain_din, sm_coef_gain_en, sm_coef_buffer_addr, sm_coef_buffer_din, sm_coef_buffer_we] = plb_memmap(wrDBus, bankAddr, linearAddr, RNWReg, addrAck, sm_coef_update, sm_coef_gain, sm_coef_buffer)
      | 
      | 
      | % connvert the input data to UFix_32_0 (the bus data type)
      | % 'From Register' blocks
      | % 'To Register' blocks
      | 
      | % sm_coef_update_dout = xfix({xlUnsigned, 32, 0}, 0);
      | sm_coef_update_dout = xl_force(sm_coef_update, xlUnsigned, 0);
      | 
      | % sm_coef_gain_dout = xfix({xlUnsigned, 32, 0}, 0);
      | sm_coef_gain_dout = xl_force(sm_coef_gain, xlUnsigned, 0);
      | 
      | 
      | % 'From FIFO' blocks
      | % 'To FIFO' blocks
      | % 'Shared Memory' blocks
      | % coef_buffer_bus = xfix({xlUnsigned, 32, 0}, 0);
      | sm_coef_buffer_bus = xl_force(sm_coef_buffer, xlUnsigned, 0);
      | 
      | 
      | % 'dout' ports of 'From Register' blocks
      | 
      | % registered register mux output
      | persistent reg_bank_out_reg; reg_bank_out_reg = xl_state(0, {xlUnsigned, 32, 0});
      | reg_bank_out = reg_bank_out_reg;
      | 
      | if linearAddr == 0
      |     reg_bank_out_reg = sm_coef_update_dout;
      | elseif linearAddr == 1
      |     reg_bank_out_reg = sm_coef_gain_dout;
      | 
      | end
      | 
      | 
      | % 'From FIFO' and 'To FIFO' blocks
      | 
      | 
      | 
      | 
      | 
      | opCode = xl_concat(addrAck, RNWReg, bankAddr, linearAddr);
      | 
      | % 'Shared Memory' blocks
      | 
      | sm_coef_buffer_sel = true;
      | 
      | % registered Shared Memory mux output
      | persistent ram_bank_out_reg; ram_bank_out_reg = xl_state(0, {xlUnsigned, 32, 0});
      | ram_bank_out = ram_bank_out_reg;
      | if sm_coef_buffer_sel
      |     ram_bank_out_reg = sm_coef_buffer_bus;
      | end
      | 
      | % 'din' ports of 'Shared Memory' blocks
      | sm_coef_buffer_din = xl_force(xl_slice(wrDBus, 7 - 1, 0), ...
      |                                  xlSigned, ...
      |                                  0);
      | 
      | 
      | % 'we' ports of 'Shared Memory' blocks
      | persistent sm_coef_buffer_we_reg; sm_coef_buffer_we_reg = xl_state(false, {xlBoolean});
      | sm_coef_buffer_we = sm_coef_buffer_we_reg;
      | opCode_sm_coef_buffer = xl_concat(addrAck, RNWReg, bankAddr);
      | if opCode_sm_coef_buffer == xfix({xlUnsigned, 4, 0}, 8);
      |     sm_coef_buffer_we_reg = true;
      | else
      |     sm_coef_buffer_we_reg = false;
      | end
      | 
      | 
      | % 'addr' ports of 'Shared Memory' blocks
      | persistent sm_coef_buffer_addr_reg; 
      | sm_coef_buffer_addr_reg = xl_state(0, {xlUnsigned, 5, 0});
      | sm_coef_buffer_addr = sm_coef_buffer_addr_reg;
      | sm_coef_buffer_addr_reg = linearAddr;
      | 
      | 
      | % 're' ports of 'From FIFO' blocks
      | 
      | 
      | % 'en' ports of 'To Register' blocks
      | if opCode == xl_concat(xfix({xlUnsigned, 4, 0}, 10), ...
      |                        xfix({xlUnsigned, xl_nbits(linearAddr), 0}, 0))
      |     sm_coef_update_en = true;
      | else
      |     sm_coef_update_en = false;
      | end
      | if opCode == xl_concat(xfix({xlUnsigned, 4, 0}, 10), ...
      |                        xfix({xlUnsigned, xl_nbits(linearAddr), 0}, 1))
      |     sm_coef_gain_en = true;
      | else
      |     sm_coef_gain_en = false;
      | end
      | 
      | 
      | % 'din' ports of 'To FIFO' blocks
      | 
      | 
      | % 'we' ports of 'To FIFO' blocks
      | 
      | 
      | % 'din' ports of 'To Register' blocks
      | sm_coef_update_din = xl_force(xl_slice(wrDBus, 1 - 1, 0), ...
      |                                  xlUnsigned, ...
      |                                  0);
      | sm_coef_gain_din = xl_force(xl_slice(wrDBus, 20 - 1, 0), ...
      |                                  xlUnsigned, ...
      |                                  17);
      | 
      | 
      | persistent read_bank_out_reg; read_bank_out_reg = xl_state(0, {xlUnsigned, 32, 0});
      | read_bank_out = read_bank_out_reg;
      | 
      | persistent bankAddr_reg; bankAddr_reg = xl_state(0, bankAddr);
      | 
      | if bankAddr_reg == 0
      |     % Bank 0: Shared Memories
      |     read_bank_out_reg = ram_bank_out;
      | elseif bankAddr_reg == 1
      |     % Bank 1: From/To FIFOs
      |     read_bank_out_reg =  0;
      | elseif bankAddr_reg == 2
      |     % Bank 2: From/To Registers
      |     read_bank_out_reg = reg_bank_out;
      | elseif bankAddr_reg == 3
      |     % Bank 3: Configuration Registers
      |     read_bank_out_reg = 0;
      | end
      | 
      | bankAddr_reg = bankAddr;
  sg_plb_addrpref : xbsIndex_r4/Gateway In  gui_display_data_type=Fixed-point  arith_type=Unsigned  n_bits=20  bin_pt=0  preci_type=Single  exp_width=8  frac_width=24  quantization="Round  (unbiased: +/- Inf)"  overflow=Saturate  period=xlGetNormalizedPeriod()  dbl_ovrd=off  timing_constraint=None  locs_specified=off  LOCs={}  hdl_port=on  block_type=gatewayin
      settings: infoedit="Gateway in block.  Converts inputs of type Simulink integer, double and fixed point to  Xilinx fixed point or floating-point data type.<br><br>Hardware notes:  In hardware these blocks become top level input ports."  sginterface={'Xilinx'=>{'jtaghwcosim'=>{'non_memory_mapped_port'=>'sg_plb_addrpref'}},'iopad'=>{'constraint'=>'#'}}
  wires:
  plb_decode/2 -> plb_memmap/5, Sl_addrAck/1  "Sl_addrAck"
  plb_decode/4 -> Sl_wrDAck/1, Sl_wrComp/1  "Sl_wrDAck"
  plb_memmap/8 -> Shared Memory/3  "coef_buffer_we"
  plb_memmap/7 -> Shared Memory/2  "coef_buffer_din"
  plb_memmap/6 -> Shared Memory/1  "coef_buffer_addr"
  plb_memmap/5 -> To Register1/2  "coef_gain_en"
  plb_memmap/4 -> To Register1/1  "coef_gain_din"
  plb_memmap/3 -> To Register/2  "coef_update_en"
  plb_memmap/2 -> To Register/1  "coef_update_din"
  plb_memmap/1 -> plb_decode/6  "rdData"
  Shared Memory/1 -> plb_memmap/8  "coef_buffer_dout"
  To Register1/1 -> plb_memmap/7  "coef_gain_dout"
  To Register/1 -> plb_memmap/6  "coef_update_dout"
  plb_decode/6 -> plb_memmap/4  "RNWReg"
  plb_decode/9 -> plb_memmap/3  "linearAddr"
  plb_decode/5 -> plb_memmap/2  "bankAddr"
  plb_decode/1 -> plb_memmap/1  "wrDBusReg"
  plb_decode/8 -> Sl_rdDBus/1  "Sl_rdDBus"
  plb_decode/7 -> Sl_rdDAck/1  "Sl_rdDAck"
  plb_decode/3 -> Sl_rdComp/1  "Sl_rdComp"
  sg_plb_addrpref/1 -> plb_decode/7  "addrPref"
  PLB_wrDBus/1 -> plb_decode/5  "PLB_wrDBus"
  PLB_RNW/1 -> plb_decode/4  "PLB_RNW"
  PLB_PAValid/1 -> plb_decode/3  "PLB_PAValid"
  PLB_ABus/1 -> plb_decode/2  "PLB_ABus"
  SPLB_Rst/1 -> plb_decode/1  "SPLB_Rst"
  Constant6/1 -> sg_plb_addrpref/1
  Constant5/1 -> Sl_wait/1  "Sl_wait"
  Constant4/1 -> PLB_wrDBus/1
  Constant3/1 -> PLB_RNW/1
  Constant2/1 -> PLB_PAValid/1
  Constant1/1 -> PLB_ABus/1
  Constant/1 -> SPLB_Rst/1
  Sl_wrComp/1 -> Terminator6/1
  Sl_wrDAck/1 -> Terminator5/1
  Sl_wait/1 -> Terminator4/1
  Sl_rdDBus/1 -> Terminator3/1
  Sl_rdDAck/1 -> Terminator2/1
  Sl_rdComp/1 -> Terminator1/1
  Sl_addrAck/1 -> Terminator/1

== system sg_2d_fir/sg_2d_fir/5x5_Filters/Blue_Filter ==
  Addr : Inport
  Din : Inport  Port=2
  Load : Inport  Port=3
  Coef : Inport  Port=4
  Gain : Inport  Port=5
  5x5_Filter : Subsystem  mask(5x5 Filter){maskNum=Gaussian, coef_n_bits=7, coef_bin_pt=0, gain_n_bits=20, gain_bin_pt=17, smpl_n_bits=8, smpl_bin_pt=0, smpl_period=1, maskCoef=0, maskDiv=0}
      mask prompts: maskNum "5x5 Mask"; coef_n_bits "Coefficient Width"; coef_bin_pt "Coefficient Binary Point"; gain_n_bits "Gain Width"; gain_bin_pt "Gain Binary Point"; smpl_n_bits "Number of Bits per Input Sample"; smpl_bin_pt "Binary Point for Input Samples"; smpl_period "Sample Period"; maskCoef "Mask Value"; maskDiv "Mask Division"
      mask help: The 5x5 Filter block is implemented using 5 n-tap MAC FIR Filters. Nine different 2-D filters have been provided to filter grayscale images.
      mask init:
      | % [bg,fg] = xlcmap('XBlock',0);
      | % iPos = get_param(gcb,'Position');
      | % iWidth=iPos(3)-iPos(1); iHeight=iPos(4)-iPos(2);
      | % iCx=iWidth/2;
      | % iCy=iHeight/2;
      | % [logoX, logoY] = xlogo(iPos);
      | 
      | % Different 5x5 Filters 
      | %  by default identity is used
      | 
      | identity = [ 0  0  0  0 0; ...
      |              0  0  0  0 0; ...
      |              0  0  1  0 0; ...
      |              0  0  0  0 0; ...
      |              0  0  0  0 0];
      | %identityDiv = 1;
      | identityDiv = 131072;
      | 
      | edge = [ 0  0  0  0 0; ...
      |          0 -1 -1 -1 0; ...
      |          0 -1  8 -1 0; ...
      |          0 -1 -1 -1 0; ...
      |          0  0  0  0 0];
      | %edgeDiv = 1;
      | edgeDiv = 131072;
      | 
      | sobelX = [ 0  0  0  0 0; ...
      |            0 -1  0  1 0; ...
      |            0 -2  0  2 0; ...
      |            0 -1  0  1 0; ...
      |            0  0  0  0 0];
      | %sobelXDiv = 1;
      | sobelXDiv = 131072;
      | 
      | sobelY = [ 0  0  0  0 0; ...
      |            0  1  2  1 0; ...
      |            0  0  0  0 0; ...
      |            0 -1 -2 -1 0; ...
      |            0  0  0  0 0];
      | %sobelYDiv = 1;
      | sobelYDiv = 131072;
      | 
      | sobelXY = [ 0  0  0  0 0; ...
      |             0  0 -1 -1 0; ...
      |             0  1  0 -1 0; ...
      |             0  1  1  0 0; ...
      |             0  0  0  0 0];
      | %sobelXYDiv = 1;
      | sobelXYDiv = 131072;
      | 
      | blur = [ 1  1  1  1 1; ...
      |          1  0  0  0 1; ...
      |          1  0  0  0 1; ...
      |          1  0  0  0 1; ...
      |          1  1  1  1 1];
      | %blurDiv = 1/16;
      | blurDiv = 8192;
      | 
      | smooth = [ 1  1  1  1 1; ...
      |            1  5  5  5 1; ...
      |            1  5 44  5 1; ...
      |            1  5  5  5 1; ...
      |            1  1  1  1 1];
      | %smoothDiv = 1/100;
      | smoothDiv = 1310;
      | 
      | sharpen = [ 0  0  0  0 0; ...
      |             0 -2 -2 -2 0; ...
      |             0 -2 32 -2 0; ...
      |             0 -2 -2 -2 0; ...
      |             0  0  0  0 0];
      | %sharpenDiv = 1/16;
      | sharpenDiv = 8192;
      | 
      | gaussian = [1 1 2 1 1; ...
      |             1 2 4 2 1; ...
      |             2 4 8 4 2; ...
      |             1 2 4 2 1; ...
      |             1 1 2 1 1];
      | %gaussianDiv = 1/52;
      | gaussianDiv = 2521;
      | 
      | maskCoef = zeros(5,5,5);
      | maskCoef(:,:,1) = identity;
      | maskCoef(:,:,2) = edge;
      | maskCoef(:,:,3) = sobelX;
      | maskCoef(:,:,4) = sobelY;
      | maskCoef(:,:,5) = sobelXY;
      | maskCoef(:,:,6) = blur;
      | maskCoef(:,:,7) = smooth;
      | maskCoef(:,:,8) = sharpen;
      | maskCoef(:,:,9) = gaussian;
      | 
      | 
      | maskDiv = [identityDiv edgeDiv sobelXDiv sobelYDiv sobelXYDiv blurDiv smoothDiv sharpenDiv gaussianDiv];
      mask StyleString: popup(Identity|Edge|Sobel X|Sobel Y|Sobel X-Y|Blur|Smooth|Sharpen|Gaussian),edit,edit,edit,edit,edit,edit,edit,edit,edit
  Line_Buffer : Subsystem
  Dout : Outport
  wires:
  5x5_Filter/1(Dout) -> Dout/1  "dout"
  Line_Buffer/1(l1) -> 5x5_Filter/1(Line1)  "l1"
  Line_Buffer/2(l2) -> 5x5_Filter/2(Line2)  "l2"
  Line_Buffer/3(l3) -> 5x5_Filter/3(Line3)  "l3"
  Line_Buffer/4(l4) -> 5x5_Filter/4(Line4)  "l4"
  Line_Buffer/5(l5) -> 5x5_Filter/5(Line5)  "l5"
  Din/1 -> Line_Buffer/2(data)  "din"
  Load/1 -> 5x5_Filter/6(load)
  Coef/1 -> 5x5_Filter/7(coef)
  Gain/1 -> 5x5_Filter/8(gain)
  Addr/1 -> Line_Buffer/1(addr)  "addr"

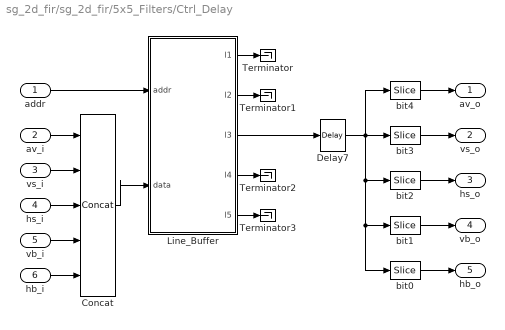
== system sg_2d_fir/sg_2d_fir/5x5_Filters/Ctrl_Delay ==
  addr : Inport
  av_i : Inport  Port=2
  vs_i : Inport  Port=3
  hs_i : Inport  Port=4
  vb_i : Inport  Port=5
  hb_i : Inport  Port=6
  Concat : xbsIndex_r4/Concat  num_inputs=5  dbl_ovrd=off  block_type=concat
      settings: block_version=9.1.01
  Delay7 : xbsIndex_r4/Delay  rst=off  infoeditControl=Selection of Reset will increase slice count due to use of real FFs and instead of SRLs  en=off  latency=26  dbl_ovrd=off  reg_retiming=on  block_type=delay
      settings: infoedit="Delay line having  configurable length.<P><P>Hardware notes: A delay line is a chain, each link of which is an SRL16 followed by a flip-flop. If register retiming is enabled, the delay line is a chain of flip-flops."  xl_area=[0, 0, 0, 0, 0, 0, 0]  block_version=VER_STRING_GOES_HERE
  Line_Buffer : Subsystem
  Terminator{,1..3} (4 alike) : Terminator
  bit0 : xbsIndex_r4/Slice  nbits=1  boolean_output=off  mode=Lower Bit Location + Width  bit1=0  base1=MSB of Input  bit0=0  base0=LSB of Input  dbl_ovrd=off  block_type=slice
      settings: infoedit="Extracts a given range of bits from each input sample and presents it at the output.  The output type is ordinarily unsigned with binary point at zero, but can be Boolean when the slice is one bit wide.<P><P>Hardware notes: In hardware this block costs nothing."  block_version=9.1.01
  bit1 : xbsIndex_r4/Slice  nbits=1  boolean_output=off  mode=Lower Bit Location + Width  bit1=0  base1=MSB of Input  bit0=1  base0=LSB of Input  dbl_ovrd=off  block_type=slice
      settings: block_version=9.1.01
  bit2 : xbsIndex_r4/Slice  nbits=1  boolean_output=off  mode=Lower Bit Location + Width  bit1=0  base1=MSB of Input  bit0=2  base0=LSB of Input  dbl_ovrd=off  block_type=slice
      settings: block_version=9.1.01
  bit3 : xbsIndex_r4/Slice  nbits=1  boolean_output=off  mode=Lower Bit Location + Width  bit1=0  base1=MSB of Input  bit0=3  base0=LSB of Input  dbl_ovrd=off  block_type=slice
      settings: block_version=9.1.01
  bit4 : xbsIndex_r4/Slice  nbits=1  boolean_output=off  mode=Lower Bit Location + Width  bit1=0  base1=MSB of Input  bit0=4  base0=LSB of Input  dbl_ovrd=off  block_type=slice
      settings: block_version=9.1.01
  av_o : Outport
  vs_o : Outport  Port=2
  hs_o : Outport  Port=3
  vb_o : Outport  Port=4
  hb_o : Outport  Port=5
  wires:
  Line_Buffer/3(l3) -> Delay7/1
  addr/1 -> Line_Buffer/1(addr)
  Line_Buffer/1(l1) -> Terminator/1
  Line_Buffer/2(l2) -> Terminator1/1
  Line_Buffer/4(l4) -> Terminator2/1
  Line_Buffer/5(l5) -> Terminator3/1
  Concat/1 -> Line_Buffer/2(data)
  av_i/1 -> Concat/1
  vs_i/1 -> Concat/2
  hs_i/1 -> Concat/3
  Delay7/1 -> bit3/1, bit4/1, bit2/1, bit1/1, bit0/1
  bit4/1 -> av_o/1
  bit3/1 -> vs_o/1
  bit2/1 -> hs_o/1
  vb_i/1 -> Concat/4
  hb_i/1 -> Concat/5
  bit1/1 -> vb_o/1
  bit0/1 -> hb_o/1
